simulink model "simudownlink"  (R2019b)
settings: Solver=VariableStepDiscrete  StartTime=0.0  StopTime=Inf  MaxStep=0.1  RelTol=1e-3
undefined symbols (not defined in the file or in its folder): paramRFSatLink
libraries: commrflib2 x2, commdigbbndfm2 x2, commfilt2 x2, impairlib x1, commsink2 x1, commchan3 x1, commrandsrc3 x1, commdigbbndcpm2 x1
settings Model: Creator=russe  LastModifiedBy=russe

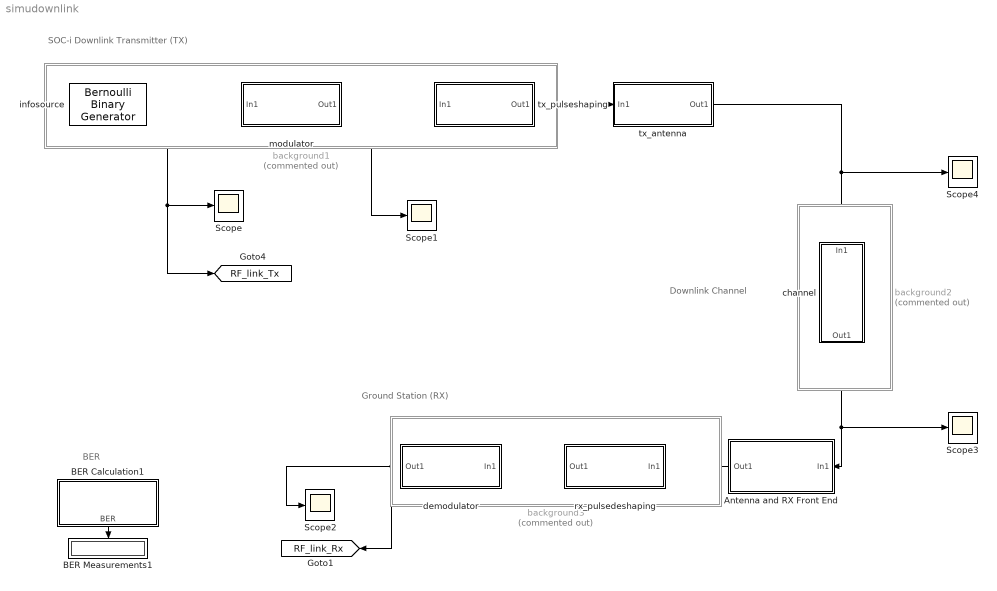
== system simudownlink ==
  note: SOC-i Downlink Transmitter (TX)
  note: Downlink Channel
  note: Ground Station (RX)
  note: BER
  Antenna and RX Front End : Subsystem
      mask Display: disp('Antenna and\nRX Front End')
  BER Calculation1 : Subsystem
      mask Display: disp('Display Complete\nBit Error Rate\nInformation');
  BER Measurements1 : Display
      settings: Format=short_e
  Scope{,1..4} (5 alike) : Scope
  background1 : Subsystem  Commented=on
      mask Display: disp('')
  background2 : Subsystem  Commented=on
      mask Display: disp('')
  background3 : Subsystem  Commented=on
      mask Display: disp('')
  channel : Subsystem
  demodulator : Subsystem
  "infosource " : commrandsrc3/Bernoulli Binary Generator  ProbabilityOfZero=0.5  SeedSource=Auto  Seed=0  SampleTime=1/(4*9600)  SamplesPerFrame=4  OutputDataType=double  SimulateUsing=Interpreted execution
      settings: SourceProductName=Communications Toolbox
  modulator : Subsystem
  rx_pulsedeshaping : Subsystem
  tx_antenna : Subsystem
  tx_pulseshaping : Subsystem
  tag scope: RF_link_Rx=global, RF_link_Tx=global
  wires:
  "infosource "/1 -> modulator/1(In1), [RF_link_Tx], Scope/1
  demodulator/1(Out1) -> Scope2/1, [RF_link_Rx]
  modulator/1(Out1) -> tx_pulseshaping/1(In1), Scope1/1
  BER Calculation1/1(BER) -> BER Measurements1/1
  channel/1(Out1) -> Antenna and RX Front End/1(In1), Scope3/1
  tx_antenna/1(Out1) -> Scope4/1, channel/1(In1)
  Antenna and RX Front End/1(Out1) -> rx_pulsedeshaping/1(In1)
  rx_pulsedeshaping/1(Out1) -> demodulator/1(In1)
  tx_pulseshaping/1(Out1) -> tx_antenna/1(In1)

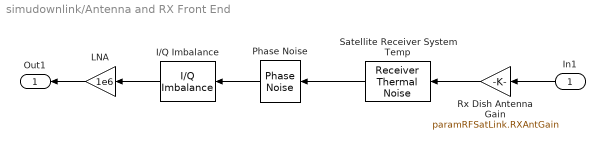
== system simudownlink/Antenna and RX Front End ==
  In1 : Inport
  I/Q Imbalance : commrflib2/I//Q Imbalance  ampImbal=paramRFSatLink.IQImbal(1)  phsImbal=paramRFSatLink.IQImbal(2)  Idc=paramRFSatLink.IQImbal(3)  Qdc=paramRFSatLink.IQImbal(4)
      settings: SourceProductName=Communications Toolbox  SourceProductBaseCode=CM
  LNA : Gain  Gain=1e6
  Phase Noise : impairlib/Phase Noise  Level=paramRFSatLink.PhaseNoise  FrequencyOffset=100  SampleRate=2e5  RandomStream=mt19937ar with seed  Seed=2137  SimulateUsing=Interpreted execution
      settings: SourceProductName=SerDes Toolbox  SourceProductBaseCode=SX
  Rx Dish Antenna Gain : Gain  Gain=paramRFSatLink.RXAntGain  SaturateOnIntegerOverflow=on  OutDataTypeStr=Inherit: Same as input  ParamDataTypeStr=Inherit: Same as input
  Satellite Receiver System Temp : commrflib2/Receiver Thermal Noise  method=Noise temperature  ntemp=paramRFSatLink.RXTemp  nfigure=20  nfactor=2  add290KAntennaNoise=off  seed=67987
      settings: SourceProductName=Communications Toolbox  SourceProductBaseCode=CM
  Out1 : Outport  VectorParamsAs1DForOutWhenUnconnected=off
  wires:
  LNA/1 -> Out1/1
  Phase Noise/1 -> I/Q Imbalance/1
  Satellite Receiver System Temp/1 -> Phase Noise/1
  In1/1 -> Rx Dish Antenna Gain/1
  I/Q Imbalance/1 -> LNA/1
  Rx Dish Antenna Gain/1 -> Satellite Receiver System Temp/1

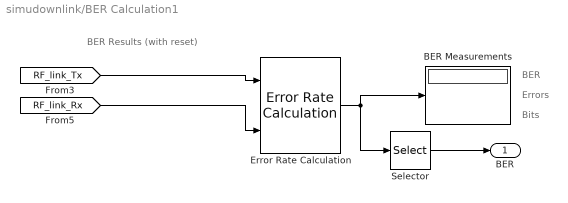
== system simudownlink/BER Calculation1 ==
  note: BER Results (with reset)
  note: Bits
  note: Errors
  note: BER
  BER Measurements : Display
  Error Rate Calculation : commsink2/Error Rate Calculation  N=24  st_delay=0  cp_mode=Entire frame  subframe=[]  PMode=Port  WsName=ErrorVec  RsMode2=off  stop=off  numErr=200  maxBits=1e6
      settings: SourceProductName=Communications Toolbox
  Selector : Selector  InputPortWidth=3  IndexOptions=Index vector (dialog)  Indices=[1]  OutputSizes=1
  BER : Outport  VectorParamsAs1DForOutWhenUnconnected=off
  wires:
  [RF_link_Tx] -> Error Rate Calculation/1
  Selector/1 -> BER/1
  Error Rate Calculation/1 -> BER Measurements/1, Selector/1
  [RF_link_Rx] -> Error Rate Calculation/2

== system simudownlink/background1 ==

== system simudownlink/background2 ==

== system simudownlink/background3 ==

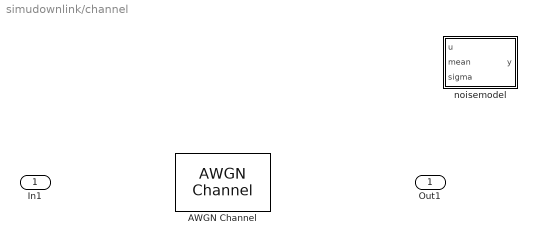
== system simudownlink/channel ==
  In1 : Inport
  AWGN Channel : commchan3/AWGN Channel  InputProcessing=Columns as channels (frame based)  seed=67  noiseMode="Signal to noise ratio  (Eb/No)"  EbNodB=10  EsNodB=10  SNRdB=10  bitsPerSym=2  Ps=1  Tsym=2/9600  variance=1
      settings: SourceProductName=Communications Toolbox
  noisemodel : MATLAB Function  TreatAsAtomicUnit=on
  Out1 : Outport

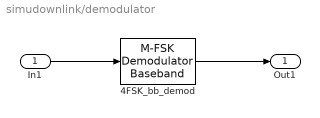
== system simudownlink/demodulator ==
  In1 : Inport
  4FSK_bb_demod : commdigbbndfm2/M-FSK Demodulator Baseband  M=4  OutType=Bit  Dec=Gray  freqSep=1  numSamp=1  RateOptions=Enforce single-rate processing  outDataType=double
      settings: SourceProductName=Communications Toolbox  SourceProductBaseCode=CM
  Out1 : Outport
  wires:
  In1/1 -> 4FSK_bb_demod/1
  4FSK_bb_demod/1 -> Out1/1

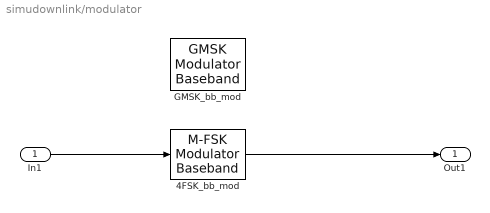
== system simudownlink/modulator ==
  In1 : Inport
  " 4FSK_bb_mod" : commdigbbndfm2/M-FSK Modulator Baseband  M=4  InType=Bit  Enc=Gray  freqSep=1  phaseType=Continuous  numSamp=1  RateOptions=Enforce single-rate processing  outDataType=double
      settings: SourceProductName=Communications Toolbox
  GMSK_bb_mod : commdigbbndcpm2/GMSK Modulator Baseband  inputType=Integer  BT=.3  pulseLength=4  preHistory=1  phaseOffset=0  samplesPerSymbol=8  RateOptions=Enforce single-rate processing  outDataType=double
      settings: SourceProductName=Communications Toolbox  SourceProductBaseCode=CM
  Out1 : Outport
  wires:
  In1/1 -> " 4FSK_bb_mod"/1
  " 4FSK_bb_mod"/1 -> Out1/1

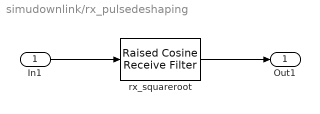
== system simudownlink/rx_pulsedeshaping ==
  In1 : Inport
  rx_squareroot : commfilt2/Raised Cosine Receive Filter  filtType=Square root  R=0.2  filtSpan=16  N=2  downFactor=2  downOffset=0  filterGain=1  InputProcessing=Columns as channels (frame based)  RateOptions=Enforce single-rate processing  framing=Mute  checkCoeff=off  variableName=rcRxFilt  currentFiltSpan=16  D=(16)/2  inputOffset=0  sampMode=Mute  saveAsFlag=0  rateMode=Downsampling  checkGain=Normalized  launchFVT=on  roundingMode=Floor  overflowMode=off  coeffDataTypeStr=Inherit: Same word length as input  coeffMin=[]  coeffMax=[]  coeffLastDataTypeStr=Inherit: Same word length as input  accumDataTypeStr=Inherit: Same as product output  accumLastDataTypeStr=Inherit: Same as product output  outputDataTypeStr=Inherit: Same as accumulator  outputMin=[]  outputMax=[]  outputLastDataTypeStr=Inherit: Same as accumulator
      settings: SourceProductName=Communications Toolbox
  Out1 : Outport
  wires:
  In1/1 -> rx_squareroot/1
  rx_squareroot/1 -> Out1/1

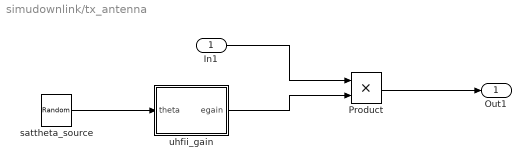
== system simudownlink/tx_antenna ==
  In1 : Inport
  Product : Product
  sattheta_source : UniformRandomNumber  Minimum=-7  Maximum=7  SampleTime=0.1
  uhfii_gain : MATLAB Function  TreatAsAtomicUnit=on
  Out1 : Outport
  wires:
  uhfii_gain/1(egain) -> Product/2
  Product/1 -> Out1/1
  sattheta_source/1 -> uhfii_gain/1(theta)
  In1/1 -> Product/1

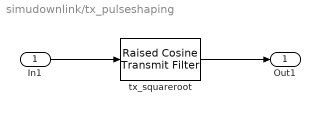
== system simudownlink/tx_pulseshaping ==
  In1 : Inport
  tx_squareroot : commfilt2/Raised Cosine Transmit Filter  filtType=Square root  R=0.2  filtSpan=16  N=2  filterGain=1  InputProcessing=Columns as channels (frame based)  RateOptions=Enforce single-rate processing  framing=Mute  checkCoeff=off  variableName=rcTxFilt  checkGain=Normalized  sampMode=Mute  saveAsFlag=0  currentFiltSpan=16  D=(16)/2  launchFVT=on  roundingMode=Floor  overflowMode=off  coeffDataTypeStr=Inherit: Same word length as input  coeffMin=[]  coeffMax=[]  coeffLastDataTypeStr=Inherit: Same word length as input  outputDataTypeStr=Inherit: Same as accumulator  outputMin=[]  outputMax=[]  outputLastDataTypeStr=Inherit: Same as accumulator
      settings: SourceProductName=Communications Toolbox
  Out1 : Outport
  wires:
  In1/1 -> tx_squareroot/1
  tx_squareroot/1 -> Out1/1

== matlab function simudownlink/tx_antenna/uhfii_gain ==
  data: theta input; egain output
function egain = satpointing(theta)
% theta - input from source model for satellite angle ([-7,7] right now)
% egain - gain of endurosat antenna due to directionality
c = .9445;
a = -9.0816*10^(-4);
egain =  a*(theta^2) + c;

== matlab function simudownlink/channel/noisemodel ==
  data: u input; y output; mean input; sigma input
function y = gaussiannoise(u,mean,sigma)
% Implement AWGN with a transparent function instead of a black box
% u is signal to add gaussian noise to
% mean is centroid (mean)
% sigma is variance
